simulink model "ParadigmPresenterStandardModel"  (R2017a)
settings: Solver=FixedStepDiscrete  StartTime=0.0  StopTime=inf  FixedStep=1/1200  RelTol=1e-3  EnableMultiTasking=on
model workspace (MAT data in the model file):
  buffer_size = 16
  cfg_native : struct (value not decoded)
  device_serial = 'HA-2011.09.08'
  number_of_channels = 161
  sample_rate = 1200
undefined symbols (not defined in the file): groupMap
libraries: gtecHighspeedLib x3
settings Model: ModifiedByFormat=g.tec  Creator=g.tec medical engineering  LastModifiedBy=g.tec
settings DataIOCC: LimitDataPoints=on  SaveFormat=Array
settings OptimizationCC: LifeSpan=inf
settings DebuggingCC: SFUnexpectedBacktrackingDiag=warning  SFNoUnconditionalDefaultTransitionDiag=warning  SFExecutionAtInitializationDiag=none
settings HardwareCC: ProdBitPerPointer=32  ProdBitPerSizeT=32  ProdBitPerPtrDiffT=32  ProdLargestAtomicFloat=None  ProdIntDivRoundTo=Undefined  ProdEndianess=Unspecified  ProdWordSize=32  ProdHWDeviceType=32-bit Generic
settings ModelReferenceCC: PropagateSignalLabelsOutOfModel=off
settings GRTTargetCC: TargetLangStandard=C89/C90 (ANSI)  GeneratePreprocessorConditionals=Disable all
settings ConfigComp: CovMetricSettings=dw  CovHtmlReporting=on  CovSaveCumulativeToWorkspaceVar=on  CovSaveSingleToWorkspaceVar=on  CovExternalEMLEnable=off

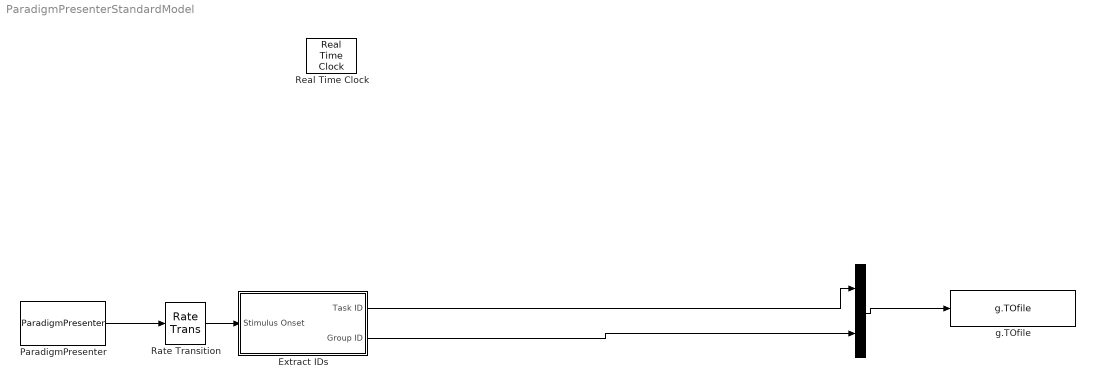
== system ParadigmPresenterStandardModel ==
  "  " : Concatenate
  Extract IDs : Subsystem
  ParadigmPresenter : gtecHighspeedLib/ParadigmPresenter  Priority=2  sharedMemoryId=0INGXDLN0L  bufferSize=000001  sampleRateOrig=001200  stimQuantizationUs=002000  paradigmRootFolder=D:\EEG_caps_comparison\MotorImagery  logLevel=1  paradigmFiles=\MotorImagery.xml
      settings: SourceProductName=g.tec Highspeed Library
  Rate Transition : RateTransition
  Real Time Clock : gtecHighspeedLib/Real Time Clock  timeprofile=off
      settings: SourceProductName=g.tec Highspeed Library
  g.TOfile : gtecHighspeedLib/g.TOfile  filename=test  varname=y  filesize=1800  blocksize=512  enable=off  save_model=off  patient_data=off  id=ID0000  firstname=John  lastname=Doe  dateofbirth=12.01.2001  sex=FEMALE  hand=MIXED  diagnosis=Diagnosis  medication=Medication Text  comments=any text ...  run=1  session=1
      settings: SourceProductName=g.tec Highspeed Library
  wires:
  "  "/1 -> g.TOfile/1
  ParadigmPresenter/1 -> Rate Transition/1
  Rate Transition/1 -> Extract IDs/1(Stimulus Onset)
  Extract IDs/1(Task ID) -> "  "/1
  Extract IDs/2(Group ID) -> "  "/2

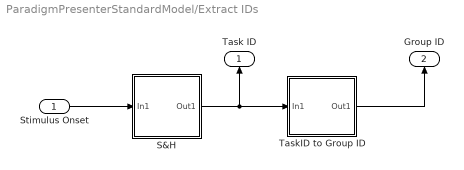
== system ParadigmPresenterStandardModel/Extract IDs ==
  Stimulus Onset : Inport
  S&H : Subsystem
  TaskID to Group ID : Subsystem  InitFcn=|
      | try
      |   taskInfo = evalin('base','taskInfo');
      |   groupMap = taskInfo.Group;
      | catch ME
      |   clear ME;
      |   error('No paradigm loaded!');
      | end
  Task ID : Outport
  Group ID : Outport  Port=2
  wires:
  TaskID to Group ID/1(Out1) -> Group ID/1
  S&H/1(Out1) -> TaskID to Group ID/1(In1), Task ID/1
  Stimulus Onset/1 -> S&H/1(In1)

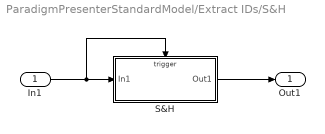
== system ParadigmPresenterStandardModel/Extract IDs/S&H ==
  In1 : Inport
  S&H : Subsystem  TreatAsAtomicUnit=on
  Out1 : Outport
  wires:
  In1/1 -> S&H/Trigger, S&H/1(In1)
  S&H/1(Out1) -> Out1/1

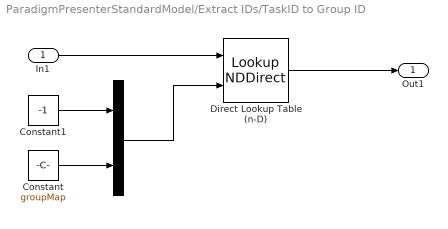
== system ParadigmPresenterStandardModel/Extract IDs/TaskID to Group ID ==
  In1 : Inport
  " " : Concatenate
  Constant : Constant  Value=groupMap
  Constant1 : Constant  Value=-1
  Direct Lookup Table (n-D) : LookupNDDirect  NumberOfTableDimensions=1  TableIsInput=on  Table=[4 5 ;16 19 ]  DiagnosticForOutOfRangeInput=Error
  Out1 : Outport
  wires:
  Direct Lookup Table (n-D)/1 -> Out1/1
  In1/1 -> Direct Lookup Table (n-D)/1
  Constant/1 -> " "/2
  Constant1/1 -> " "/1
  " "/1 -> Direct Lookup Table (n-D)/2

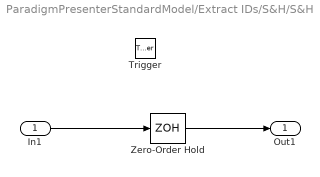
== system ParadigmPresenterStandardModel/Extract IDs/S&H/S&H ==
  In1 : Inport
  Trigger : TriggerPort  VariantControl=Variant
  Zero-Order Hold : ZeroOrderHold  SampleTime=-1
  Out1 : Outport
  wires:
  In1/1 -> Zero-Order Hold/1
  Zero-Order Hold/1 -> Out1/1
